simulink model "test_MartFracTransf_03_paper"  (Simulink 7.1)
settings: Solver=ode23tb  StartTime=0.0  StopTime=1  FixedStep=1e-6  MaxStep=1e-4  RelTol=1e-3
settings Model: Creator=Vagner  LastModifiedBy=Vagner
settings DebuggingCC: AlgebraicLoopMsg=none  SolverPrmCheckMsg=none

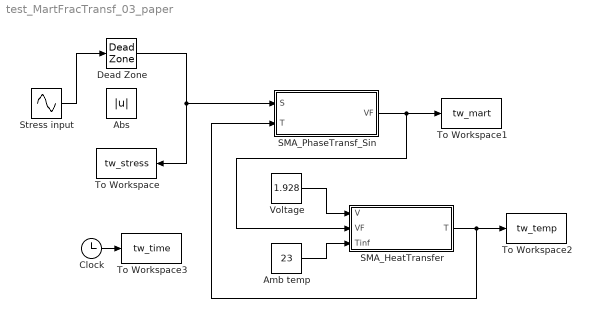
== system test_MartFracTransf_03_paper ==
  Abs : Abs  OutDataType=sfix(16)  OutScaling=2^0
  Amb temp : Constant  Value=23  OutDataType=sfix(16)  OutScaling=2^0
  Clock : Clock
      settings: Decimation=10
  Dead Zone : DeadZone  LowerValue=-inf  UpperValue=0  SaturateOnIntegerOverflow=on
  SMA_HeatTransfer : Subsystem  mask{varm=1.18e-3, varL=6025, varCp=350, varRA=0.7246, varRM=0.8197, varhc=150, varAc=977e-6, varT0=58.0049}
      mask prompts: varm "Spring mass [kg]"; varL "Latent heat [J / kg degC]"; varCp "Specific heat [J / kg degC]"; varRA "Electrical resistance of austenite [Ohm]"; varRM "Electrical resistance of martensite [Ohm]"; varhc "Convective heat transfer coefficient [J / m^2 degC s]"; varAc "Spring circunferential area [m^2]"; varT0 "Spring initial temperature [degC]"
      mask help: Mask parameters are some of the coefficients of equation (17) in Hadi et al. (2010). Commonly varying parameters are provided by input ports.
      mask init:
      | % when 'OK' or 'Apply' is clicked.
      | 
      | Hadi10_Temperature_InitMask(gcb);
      mask Help:
      | m: spring mass
      | L: latent heat
      | Cp: specific heat
      | RA: resistance in fully austenitic phase
      | RM: resistance in fully martensitic phase
      | hc: convective heat transfer coefficient
      | Ac: spring circunferential area
      | T0: spring initial temperature
      | 
      | Inputs:
      | V: voltage
      | VF: martensite volumetric fraction
      | Tinf: ambient temperature
      | 
      | Output:
      | T: spring temperature
      mask CallbackString: % Hadi10_Temperature_callback('Hadi10_Temperature_varm', gcb);|% Hadi10_Temperature_callback('Hadi10_Temperature_varL', gcb);|% Hadi10_Temperature_callback('Hadi10_Temperature_varCp', gcb);|% Hadi10_Temperature_callback('Hadi10_Temperature_varRA', gcb);|% Hadi10_Temperature_callback('Hadi10_Temperature_varRM', gcb);|% Hadi10_Temperature_callback('Hadi10_Temperature_varhc', gcb);|% Hadi10_Temperature_callback('Hadi10_Temperature_varAc', gcb);|% Hadi10_Temperature_callback('Hadi10_Temperature_varT0', gcb);
  SMA_PhaseTransf_Sin : Subsystem  mask{varCM=4, varCA=6, varSsmin=100, varSfmin=170, varMs=42, varAs=43, varAf=58}
      mask prompts: varCM "Forward stress-temperature slope (CM)"; varCA "Reverse stress-temperature slope (CA)"; varSsmin "Minimum stress for onset of forward transformation (Ssmin)"; varSfmin "Minimum stress for completion of forward transformation (Sfmin)"; varMs "Martensite start temperature (Ms)"; varAs "Austenite start temperature (As)"; varAf "Austenite finish temperature (Af)"
      mask init:
      | % when 'OK' or 'Apply' is clicked
      | 
      | SMA_PhaseTransf_Sin_InitMask(gcb);
  Stress input : Sin  Amplitude=600  Frequency=2*pi*1  SampleTime=0
  To Workspace : ToWorkspace  VariableName=tw_stress  SampleTime=-1  SaveFormat=Array
  To Workspace1 : ToWorkspace  VariableName=tw_mart  SampleTime=-1  SaveFormat=Array
  To Workspace2 : ToWorkspace  VariableName=tw_temp  SampleTime=-1  SaveFormat=Array
  To Workspace3 : ToWorkspace  VariableName=tw_time  SampleTime=-1  SaveFormat=Array
  Voltage : Constant  Value=1.928  OutDataType=sfix(16)  OutScaling=2^0
  wires:
  SMA_PhaseTransf_Sin/1(VF) -> To Workspace1/1, SMA_HeatTransfer/2(VF)
  SMA_HeatTransfer/1(T) -> To Workspace2/1, SMA_PhaseTransf_Sin/2(T)
  Voltage/1 -> SMA_HeatTransfer/1(V)
  Amb temp/1 -> SMA_HeatTransfer/3(Tinf)
  Clock/1 -> To Workspace3/1
  Dead Zone/1 -> SMA_PhaseTransf_Sin/1(S), To Workspace/1
  Stress input/1 -> Dead Zone/1

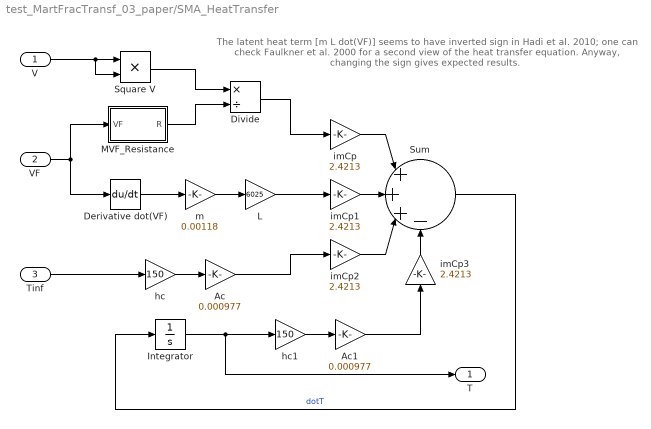
== system test_MartFracTransf_03_paper/SMA_HeatTransfer ==
  note: The latent heat term [m L dot(VF)] seems to
      | have inverted sign in Hadi et al. 2010; one
      | can check Faulkner et al. 2000 for a second
      | view of the heat transfer equation. Anyway,
      | changing the sign gives expected results.
  V : Inport  OutDataType=sfix(16)  OutScaling=2^0
  VF : Inport  Port=2  OutDataType=sfix(16)  OutScaling=2^0
  Tinf : Inport  Port=3  OutDataType=sfix(16)  OutScaling=2^0
  Ac : Gain  Gain=0.000977  ParameterDataType=sfix(16)  ParameterScaling=2^0  OutDataType=sfix(16)  OutScaling=2^0
  Ac1 : Gain  Gain=0.000977  ParameterDataType=sfix(16)  ParameterScaling=2^0  OutDataType=sfix(16)  OutScaling=2^0
  Derivative dot(VF) : Derivative
  Divide : Product  Inputs=*/  OutDataType=sfix(16)  OutScaling=2^-10
  Integrator : Integrator  InitialCondition=58.0049
  L : Gain  Gain=6025  ParameterDataType=sfix(16)  ParameterScaling=2^0  OutDataType=sfix(16)  OutScaling=2^0
  MVF_Resistance : Subsystem  mask{varRM=0.8197, varRA=0.7246}
      mask prompts: varRM "Fully-martensitic resistance [Ohm]"; varRA "Fully-austenitic resistance [Ohm]"
      mask help: Computes the electrical resistance as function of the martensitic fraction.
      mask init:
      | % when 'OK' or 'Apply' is clicked
      | 
      | MVF_Resistance_InitMask(gcb);
      mask Help:
      | DM: Fully-martensitic electrical resistance (in Ohms)
      | DA: Fully-austenitic elastic modulus (in Ohms)
      | 
      | The linear relation is assumed:
      | R = RA + VF(RM - RA)
      mask Display:
      | port_label('input', 1, 'VF');
      | port_label('output', 1, 'R');
  Square V : Product  OutDataType=sfix(16)  OutScaling=2^0  RndMeth=Zero
  Sum : Sum  Inputs=|+++-  OutDataType=sfix(16)  OutScaling=2^0
  hc : Gain  Gain=150  ParameterDataType=sfix(16)  ParameterScaling=2^0  OutDataType=sfix(16)  OutScaling=2^0
  hc1 : Gain  Gain=150  ParameterDataType=sfix(16)  ParameterScaling=2^0  OutDataType=sfix(16)  OutScaling=2^0
  imCp : Gain  Gain=2.4213  ParameterDataType=sfix(16)  ParameterScaling=2^0  OutDataType=sfix(16)  OutScaling=2^0
  imCp1 : Gain  Gain=2.4213  ParameterDataType=sfix(16)  ParameterScaling=2^0  OutDataType=sfix(16)  OutScaling=2^0
  imCp2 : Gain  Gain=2.4213  ParameterDataType=sfix(16)  ParameterScaling=2^0  OutDataType=sfix(16)  OutScaling=2^0
  imCp3 : Gain  Orientation=up  Gain=2.4213  ParameterDataType=sfix(16)  ParameterScaling=2^0  OutDataType=sfix(16)  OutScaling=2^0
  m : Gain  Gain=0.00118  ParameterDataType=sfix(16)  ParameterScaling=2^0  OutDataType=sfix(16)  OutScaling=2^0
  T : Outport  OutDataType=sfix(16)  OutScaling=2^0
  wires:
  V/1 -> Square V/1, Square V/2
  Square V/1 -> Divide/1
  MVF_Resistance/1(R) -> Divide/2
  Divide/1 -> imCp/1
  VF/1 -> Derivative dot(VF)/1, MVF_Resistance/1(VF)
  Derivative dot(VF)/1 -> m/1
  m/1 -> L/1
  L/1 -> imCp1/1
  hc/1 -> Ac/1
  Tinf/1 -> hc/1
  Ac/1 -> imCp2/1
  hc1/1 -> Ac1/1
  imCp/1 -> Sum/1
  imCp2/1 -> Sum/3
  imCp1/1 -> Sum/2
  Integrator/1 -> hc1/1, T/1
  Ac1/1 -> imCp3/1
  imCp3/1 -> Sum/4
  Sum/1 -> Integrator/1  "dotT"

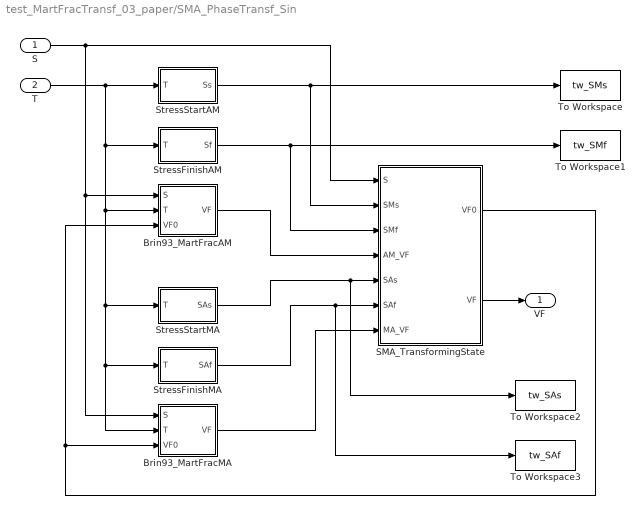
== system test_MartFracTransf_03_paper/SMA_PhaseTransf_Sin ==
  S : Inport  OutDataType=sfix(16)  OutScaling=2^0
  T : Inport  Port=2  OutDataType=sfix(16)  OutScaling=2^0
  Brin93_MartFracAM : Subsystem  mask{varSsmin=100, varSfmin=170, varCM=4, varMs=42}
      mask prompts: varSsmin "Minimum start stress"; varSfmin "Minimum finish stress"; varCM "Forward stress-temperature slope"; varMs "Martensite start temperature"
      mask init:
      | % when 'OK' or 'Apply' is clicked.
      | 
      | Brin93_MartFracAM_InitMask(gcb);
  Brin93_MartFracMA : Subsystem  mask{varCA=6, varAs=43, varAf=58}
      mask prompts: varCA "Reverse stress-temperature slope"; varAs "Austenite start temperature"; varAf "Austenite finish temperature"
      mask init:
      | % when 'OK' or 'Apply' is clicked.
      | 
      | Brin93_MartFracMA_InitMask(gcb);
  SMA_TransformingState : Subsystem
  StressFinishAM : Subsystem  mask{varCM=4, varSfmin=170, varMs=42}
      mask prompts: varCM "Forward stress-temperature slope"; varSfmin "Minimum stress for completion of transformation"; varMs "Martensite start temperature"
      mask help: Computes the critical stress for the completion of forward transformation.
      mask init:
      | % when 'OK' or 'Apply' is clicked
      | 
      | StressFinishAM_InitMask(gcb);
      mask Help:
      | Sf = Sfmin + CM * (T - Ms)
      | 
      | Sf: martensite finish stress
      | Sfmin: minimum finish stress (below Ms)
      | Ms: martensite start temperature
      | T: temperature
      mask Display:
      | port_label('input', 1, 'T');
      | port_label('output', 1, 'SMf');
  StressFinishMA : Subsystem  mask{varCA=6, varAf=58}
      mask prompts: varCA "Reverse stress-temperature slope"; varAf "Austenite finish temperature"
      mask help: Computes the critical stress for the completion of reverse transformation.
      mask init:
      | % when 'OK' or 'Apply' is clicked
      | 
      | StressFinishMA_InitMask(gcb);
      mask Help:
      | Sf = CA * (T - Af)
      | 
      | Ss: austenite finish stress
      | CA: stress-temperature slope
      | Af: austenite finish temperature
      | T: temperature
      mask Display:
      | port_label('input', 1, 'T');
      | port_label('output', 1, 'SAf');
  StressStartAM : Subsystem  mask{varCM=4, varSsmin=100, varMs=42}
      mask prompts: varCM "Forward stress-temperature slope"; varSsmin "Minimum stress for onset of transformation"; varMs "Martensite start temperature"
      mask help: Computes the critical stress for the onset of forward transformation.
      mask init:
      | % when 'OK' or 'Apply' is clicked
      | 
      | StressStartAM_InitMask(gcb);
      mask Help:
      | Ss = Ssmin + CM * (T - Ms)
      | 
      | Ss: martensite start stress
      | Ssmin: minimum start stress (below Ms)
      | Ms: martensite start temperature
      | T: temperature
      mask Display:
      | port_label('input', 1, 'T');
      | port_label('output', 1, 'SMs');
  StressStartMA : Subsystem  mask{varCA=6, varAs=43}
      mask prompts: varCA "Reverse stress-temperature slope"; varAs "Austenite start temperature"
      mask help: Computes the critical stress for the onset of reverse transformation.
      mask init:
      | % when 'OK' or 'Apply' is clicked
      | 
      | StressStartMA_InitMask(gcb);
      mask Help:
      | Ss = CA * (T - Ms)
      | 
      | Ss: austenite start stress
      | CA: stress-temperature slope
      | As: austenite start temperature
      | T: temperature
      mask Display:
      | port_label('input', 1, 'T');
      | port_label('output', 1, 'SAs');
  To Workspace : ToWorkspace  VariableName=tw_SMs  SampleTime=-1  SaveFormat=Array
  To Workspace1 : ToWorkspace  VariableName=tw_SMf  SampleTime=-1  SaveFormat=Array
  To Workspace2 : ToWorkspace  VariableName=tw_SAs  SampleTime=-1  SaveFormat=Array
  To Workspace3 : ToWorkspace  VariableName=tw_SAf  SampleTime=-1  SaveFormat=Array
  VF : Outport  OutDataType=sfix(16)  OutScaling=2^0
  wires:
  Brin93_MartFracMA/1(VF) -> SMA_TransformingState/7(MA_VF)
  Brin93_MartFracAM/1(VF) -> SMA_TransformingState/4(AM_VF)
  SMA_TransformingState/1(VF0) -> Brin93_MartFracMA/3(VF0), Brin93_MartFracAM/3(VF0)
  SMA_TransformingState/2(VF) -> VF/1
  StressFinishMA/1(SAf) -> SMA_TransformingState/6(SAf), To Workspace3/1
  StressStartMA/1(SAs) -> SMA_TransformingState/5(SAs), To Workspace2/1
  T/1 -> Brin93_MartFracAM/2(T), Brin93_MartFracMA/2(T), StressFinishMA/1(T), StressStartMA/1(T), StressFinishAM/1(T), StressStartAM/1(T)
  S/1 -> Brin93_MartFracMA/1(S), Brin93_MartFracAM/1(S), SMA_TransformingState/1(S)
  StressFinishAM/1(Sf) -> SMA_TransformingState/3(SMf), To Workspace1/1
  StressStartAM/1(Ss) -> SMA_TransformingState/2(SMs), To Workspace/1

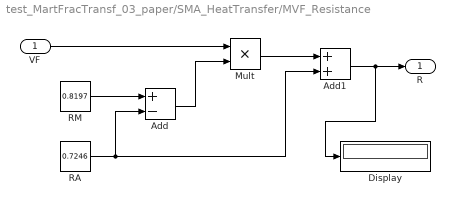
== system test_MartFracTransf_03_paper/SMA_HeatTransfer/MVF_Resistance ==
  VF : Inport  OutDataType=sfix(16)  OutScaling=2^0
  Add : Sum  Inputs=+-  OutDataType=sfix(16)  OutScaling=2^-10
  Add1 : Sum  OutDataType=sfix(16)  OutScaling=2^-10
  Display : Display
  Mult : Product  Inputs=**  OutDataType=sfix(16)  OutScaling=2^-10
  RA : Constant  Value=0.7246  OutDataType=sfix(16)  OutScaling=2^0
  RM : Constant  Value=0.8197  OutDataType=sfix(16)  OutScaling=2^0
  R : Outport  OutDataType=sfix(16)  OutScaling=2^0
  wires:
  RA/1 -> Add1/2, Add/2
  RM/1 -> Add/1
  Add1/1 -> Display/1, R/1
  Mult/1 -> Add1/1
  Add/1 -> Mult/2
  VF/1 -> Mult/1

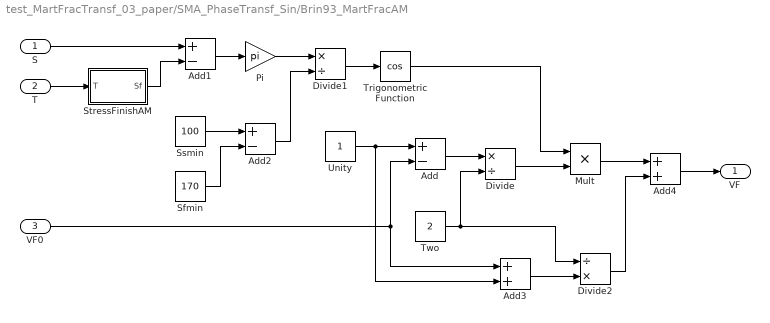
== system test_MartFracTransf_03_paper/SMA_PhaseTransf_Sin/Brin93_MartFracAM ==
  S : Inport  OutDataType=sfix(16)  OutScaling=2^0
  T : Inport  Port=2  OutDataType=sfix(16)  OutScaling=2^0
  VF0 : Inport  Port=3  OutDataType=sfix(16)  OutScaling=2^0
  Add : Sum  Inputs=+-  OutDataType=sfix(16)  OutScaling=2^-10
  Add1 : Sum  Inputs=+-  OutDataType=sfix(16)  OutScaling=2^-10
  Add2 : Sum  Inputs=+-  OutDataType=sfix(16)  OutScaling=2^-10
  Add3 : Sum  OutDataType=sfix(16)  OutScaling=2^-10
  Add4 : Sum  OutDataType=sfix(16)  OutScaling=2^-10
  Divide : Product  Inputs=*/  OutDataType=sfix(16)  OutScaling=2^-10
  Divide1 : Product  Inputs=*/  OutDataType=sfix(16)  OutScaling=2^-10
  Divide2 : Product  Inputs=/*  OutDataType=sfix(16)  OutScaling=2^-10
  Mult : Product  Inputs=**  OutDataType=sfix(16)  OutScaling=2^-10
  Pi : Gain  Gain=pi  ParameterDataType=sfix(16)  ParameterScaling=2^0  OutDataType=sfix(16)  OutScaling=2^0
  Sfmin : Constant  Value=170  OutDataType=sfix(16)  OutScaling=2^0
  Ssmin : Constant  Value=100  OutDataType=sfix(16)  OutScaling=2^0
  StressFinishAM : Subsystem  mask{varCM=4, varSfmin=170, varMs=42}
      mask prompts: varCM "Forward stress-temperature slope"; varSfmin "Minimum stress for completion of transformation"; varMs "Martensite start temperature"
      mask help: Computes the critical stress for the completion of forward transformation.
      mask init:
      | % when 'OK' or 'Apply' is clicked
      | 
      | StressFinishAM_InitMask(gcb);
      mask Help:
      | Sf = Sfmin + CM * (T - Ms)
      | 
      | Sf: martensite finish stress
      | Sfmin: minimum finish stress (below Ms)
      | Ms: martensite start temperature
      | T: temperature
      mask Display:
      | port_label('input', 1, 'T');
      | port_label('output', 1, 'SMf');
  Trigonometric Function : Trigonometry  Operator=cos
  Two : Constant  Value=2  OutDataType=sfix(16)  OutScaling=2^0
  Unity : Constant  OutDataType=sfix(16)  OutScaling=2^0
  VF : Outport  OutDataType=sfix(16)  OutScaling=2^0
  wires:
  Add3/1 -> Divide2/2
  Trigonometric Function/1 -> Mult/1
  Divide/1 -> Mult/2
  Add4/1 -> VF/1
  Divide2/1 -> Add4/2
  Mult/1 -> Add4/1
  Divide1/1 -> Trigonometric Function/1
  Add2/1 -> Divide1/2
  Sfmin/1 -> Add2/2
  Ssmin/1 -> Add2/1
  Pi/1 -> Divide1/1
  Add1/1 -> Pi/1
  StressFinishAM/1(Sf) -> Add1/2
  S/1 -> Add1/1
  Two/1 -> Divide2/1, Divide/2
  Add/1 -> Divide/1
  VF0/1 -> Add3/1, Add/2
  Unity/1 -> Add3/2, Add/1
  T/1 -> StressFinishAM/1(T)

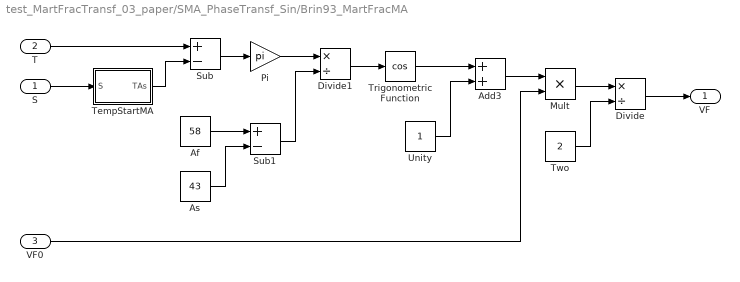
== system test_MartFracTransf_03_paper/SMA_PhaseTransf_Sin/Brin93_MartFracMA ==
  S : Inport  OutDataType=sfix(16)  OutScaling=2^0
  T : Inport  Port=2  OutDataType=sfix(16)  OutScaling=2^0
  VF0 : Inport  Port=3  OutDataType=sfix(16)  OutScaling=2^0
  Add3 : Sum  OutDataType=sfix(16)  OutScaling=2^-10
  Af : Constant  Value=58  OutDataType=sfix(16)  OutScaling=2^0
  As : Constant  Value=43  OutDataType=sfix(16)  OutScaling=2^0
  Divide : Product  Inputs=*/  OutDataType=sfix(16)  OutScaling=2^-10
  Divide1 : Product  Inputs=*/  OutDataType=sfix(16)  OutScaling=2^-10
  Mult : Product  Inputs=**  OutDataType=sfix(16)  OutScaling=2^-10
  Pi : Gain  Gain=pi  ParameterDataType=sfix(16)  ParameterScaling=2^0  OutDataType=sfix(16)  OutScaling=2^0
  Sub : Sum  Inputs=+-  OutDataType=sfix(16)  OutScaling=2^-10
  Sub1 : Sum  Inputs=+-  OutDataType=sfix(16)  OutScaling=2^-10
  TempStartMA : Subsystem  mask{varCA=6, varAs=43}
      mask prompts: varCA "Reverse stress-temperature slope"; varAs "Austenite start temperature"
      mask help: Computes the critical temperature for the onset of reverse transformation (for non-zero stress).
      mask init:
      | % when 'OK' or 'Apply' is clicked
      | 
      | TempStartMA_InitMask(gcb);
      mask Help:
      | TAs = As + S / CA
      | 
      | TAs: austenite start temperature (for S > 0)
      | CA: stress-temperature slope
      | As: austenite start temperature
      mask Display:
      | port_label('input', 1, 'S');
      | port_label('output', 1, 'TAs');
  Trigonometric Function : Trigonometry  Operator=cos
  Two : Constant  Value=2  OutDataType=sfix(16)  OutScaling=2^0
  Unity : Constant  OutDataType=sfix(16)  OutScaling=2^0
  VF : Outport  OutDataType=sfix(16)  OutScaling=2^0
  wires:
  VF0/1 -> Mult/2
  Divide/1 -> VF/1
  Add3/1 -> Mult/1
  Trigonometric Function/1 -> Add3/1
  Unity/1 -> Add3/2
  Two/1 -> Divide/2
  Mult/1 -> Divide/1
  S/1 -> TempStartMA/1(S)
  T/1 -> Sub/1
  TempStartMA/1(TAs) -> Sub/2
  Sub/1 -> Pi/1
  Pi/1 -> Divide1/1
  Af/1 -> Sub1/1
  As/1 -> Sub1/2
  Sub1/1 -> Divide1/2
  Divide1/1 -> Trigonometric Function/1

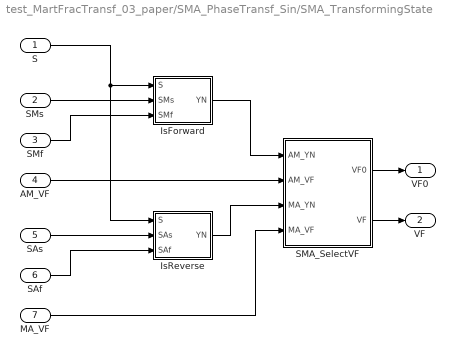
== system test_MartFracTransf_03_paper/SMA_PhaseTransf_Sin/SMA_TransformingState ==
  S : Inport
  SMs : Inport  Port=2
  SMf : Inport  Port=3
  AM_VF : Inport  Port=4
  SAs : Inport  Port=5
  SAf : Inport  Port=6
  MA_VF : Inport  Port=7
  IsForward : Subsystem
  IsReverse : Subsystem
  SMA_SelectVF : Subsystem
  VF0 : Outport
  VF : Outport  Port=2
  wires:
  MA_VF/1 -> SMA_SelectVF/4(MA_VF)
  SMA_SelectVF/2(VF) -> VF/1
  IsReverse/1(YN) -> SMA_SelectVF/3(MA_YN)
  SMA_SelectVF/1(VF0) -> VF0/1
  AM_VF/1 -> SMA_SelectVF/2(AM_VF)
  IsForward/1(YN) -> SMA_SelectVF/1(AM_YN)
  SAf/1 -> IsReverse/3(SAf)
  SAs/1 -> IsReverse/2(SAs)
  SMf/1 -> IsForward/3(SMf)
  SMs/1 -> IsForward/2(SMs)
  S/1 -> IsReverse/1(S), IsForward/1(S)

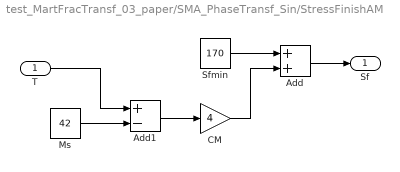
== system test_MartFracTransf_03_paper/SMA_PhaseTransf_Sin/StressFinishAM ==
  T : Inport  OutDataType=sfix(16)  OutScaling=2^0
  Add : Sum  OutDataType=sfix(16)  OutScaling=2^-10
  Add1 : Sum  Inputs=+-  OutDataType=sfix(16)  OutScaling=2^-10
  CM : Gain  Gain=4  ParameterDataType=sfix(16)  ParameterScaling=2^0  OutDataType=sfix(16)  OutScaling=2^0
  Ms : Constant  Value=42  OutDataType=sfix(16)  OutScaling=2^0
  Sfmin : Constant  Value=170  OutDataType=sfix(16)  OutScaling=2^0
  Sf : Outport  OutDataType=sfix(16)  OutScaling=2^0
  wires:
  Sfmin/1 -> Add/1
  T/1 -> Add1/1
  Ms/1 -> Add1/2
  Add1/1 -> CM/1
  CM/1 -> Add/2
  Add/1 -> Sf/1

== system test_MartFracTransf_03_paper/SMA_PhaseTransf_Sin/StressFinishMA ==
  T : Inport  OutDataType=sfix(16)  OutScaling=2^0
  Add1 : Sum  Inputs=+-  OutDataType=sfix(16)  OutScaling=2^-10
  Af : Constant  Value=58  OutDataType=sfix(16)  OutScaling=2^0
  CA : Gain  Gain=6  ParameterDataType=sfix(16)  ParameterScaling=2^0  OutDataType=sfix(16)  OutScaling=2^0
  SAf : Outport  OutDataType=sfix(16)  OutScaling=2^0
  wires:
  CA/1 -> SAf/1
  Add1/1 -> CA/1
  Af/1 -> Add1/2
  T/1 -> Add1/1

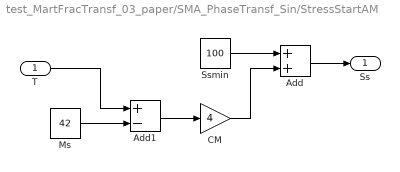
== system test_MartFracTransf_03_paper/SMA_PhaseTransf_Sin/StressStartAM ==
  T : Inport  OutDataType=sfix(16)  OutScaling=2^0
  Add : Sum  OutDataType=sfix(16)  OutScaling=2^-10
  Add1 : Sum  Inputs=+-  OutDataType=sfix(16)  OutScaling=2^-10
  CM : Gain  Gain=4  ParameterDataType=sfix(16)  ParameterScaling=2^0  OutDataType=sfix(16)  OutScaling=2^0
  Ms : Constant  Value=42  OutDataType=sfix(16)  OutScaling=2^0
  Ssmin : Constant  Value=100  OutDataType=sfix(16)  OutScaling=2^0
  Ss : Outport  OutDataType=sfix(16)  OutScaling=2^0
  wires:
  Add/1 -> Ss/1
  CM/1 -> Add/2
  Add1/1 -> CM/1
  Ms/1 -> Add1/2
  T/1 -> Add1/1
  Ssmin/1 -> Add/1

== system test_MartFracTransf_03_paper/SMA_PhaseTransf_Sin/StressStartMA ==
  T : Inport  OutDataType=sfix(16)  OutScaling=2^0
  Add1 : Sum  Inputs=+-  OutDataType=sfix(16)  OutScaling=2^-10
  As : Constant  Value=43  OutDataType=sfix(16)  OutScaling=2^0
  CA : Gain  Gain=6  ParameterDataType=sfix(16)  ParameterScaling=2^0  OutDataType=sfix(16)  OutScaling=2^0
  SAs : Outport  OutDataType=sfix(16)  OutScaling=2^0
  wires:
  CA/1 -> SAs/1
  T/1 -> Add1/1
  As/1 -> Add1/2
  Add1/1 -> CA/1

== system test_MartFracTransf_03_paper/SMA_PhaseTransf_Sin/Brin93_MartFracAM/StressFinishAM ==
  T : Inport  OutDataType=sfix(16)  OutScaling=2^0
  Add : Sum  OutDataType=sfix(16)  OutScaling=2^-10
  Add1 : Sum  Inputs=+-  OutDataType=sfix(16)  OutScaling=2^-10
  CM : Gain  Gain=4  ParameterDataType=sfix(16)  ParameterScaling=2^0  OutDataType=sfix(16)  OutScaling=2^0
  Ms : Constant  Value=42  OutDataType=sfix(16)  OutScaling=2^0
  Sfmin : Constant  Value=170  OutDataType=sfix(16)  OutScaling=2^0
  Sf : Outport  OutDataType=sfix(16)  OutScaling=2^0
  wires:
  Sfmin/1 -> Add/1
  T/1 -> Add1/1
  Ms/1 -> Add1/2
  Add1/1 -> CM/1
  CM/1 -> Add/2
  Add/1 -> Sf/1

== system test_MartFracTransf_03_paper/SMA_PhaseTransf_Sin/Brin93_MartFracMA/TempStartMA ==
  S : Inport  OutDataType=sfix(16)  OutScaling=2^0
  Add : Sum  OutDataType=sfix(16)  OutScaling=2^-10
  As : Constant  Value=43  OutDataType=sfix(16)  OutScaling=2^0
  CA : Constant  Value=6  OutDataType=sfix(16)  OutScaling=2^0
  Divide : Product  Inputs=*/  OutDataType=sfix(16)  OutScaling=2^-10
  TAs : Outport  OutDataType=sfix(16)  OutScaling=2^0
  wires:
  Add/1 -> TAs/1
  Divide/1 -> Add/1
  CA/1 -> Divide/2
  S/1 -> Divide/1
  As/1 -> Add/2

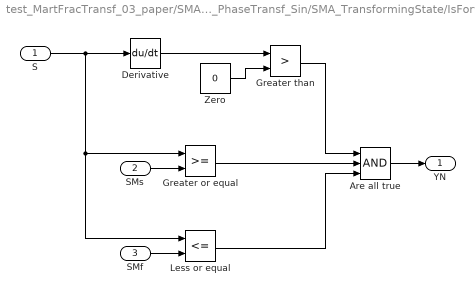
== system test_MartFracTransf_03_paper/SMA_PhaseTransf_Sin/SMA_TransformingState/IsForward ==
  S : Inport  OutDataType=sfix(16)  OutScaling=2^0
  SMs : Inport  Port=2  OutDataType=sfix(16)  OutScaling=2^0
  SMf : Inport  Port=3  OutDataType=sfix(16)  OutScaling=2^0
  Are all true : Logic  Inputs=3  AllPortsSameDT=off  OutDataTypeMode=boolean  OutDataTypeStr=boolean
  Derivative : Derivative
  Greater or equal : RelationalOperator  LogicOutDataTypeMode=boolean  OutDataTypeStr=boolean
  Greater than : RelationalOperator  Operator=>  LogicOutDataTypeMode=boolean  OutDataTypeStr=boolean
  Less or equal : RelationalOperator  Operator=<=  LogicOutDataTypeMode=boolean  OutDataTypeStr=boolean
  Zero : Constant  Value=0  OutDataType=sfix(16)  OutScaling=2^0
  YN : Outport  OutDataType=sfix(16)  OutScaling=2^0
  wires:
  Are all true/1 -> YN/1
  Less or equal/1 -> Are all true/3
  Greater or equal/1 -> Are all true/2
  Greater than/1 -> Are all true/1
  SMf/1 -> Less or equal/2
  SMs/1 -> Greater or equal/2
  Derivative/1 -> Greater than/1
  Zero/1 -> Greater than/2
  S/1 -> Less or equal/1, Greater or equal/1, Derivative/1

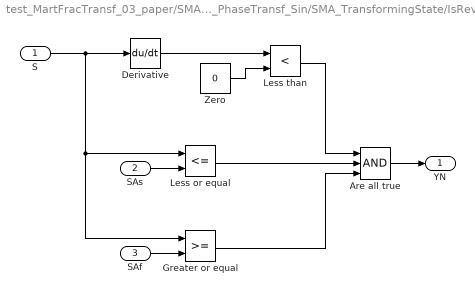
== system test_MartFracTransf_03_paper/SMA_PhaseTransf_Sin/SMA_TransformingState/IsReverse ==
  S : Inport  OutDataType=sfix(16)  OutScaling=2^0
  SAs : Inport  Port=2  OutDataType=sfix(16)  OutScaling=2^0
  SAf : Inport  Port=3  OutDataType=sfix(16)  OutScaling=2^0
  Are all true : Logic  Inputs=3  AllPortsSameDT=off  OutDataTypeMode=boolean  OutDataTypeStr=boolean
  Derivative : Derivative
  Greater or equal : RelationalOperator  LogicOutDataTypeMode=boolean  OutDataTypeStr=boolean
  Less than : RelationalOperator  Operator=<  LogicOutDataTypeMode=boolean  OutDataTypeStr=boolean
  Less or equal : RelationalOperator  Operator=<=  LogicOutDataTypeMode=boolean  OutDataTypeStr=boolean
  Zero : Constant  Value=0  OutDataType=sfix(16)  OutScaling=2^0
  YN : Outport  OutDataType=sfix(16)  OutScaling=2^0
  wires:
  S/1 -> Derivative/1, Less or equal/1, Greater or equal/1
  Zero/1 -> Less than/2
  Derivative/1 -> Less than/1
  SAs/1 -> Less or equal/2
  SAf/1 -> Greater or equal/2
  Less than/1 -> Are all true/1
  Less or equal/1 -> Are all true/2
  Greater or equal/1 -> Are all true/3
  Are all true/1 -> YN/1

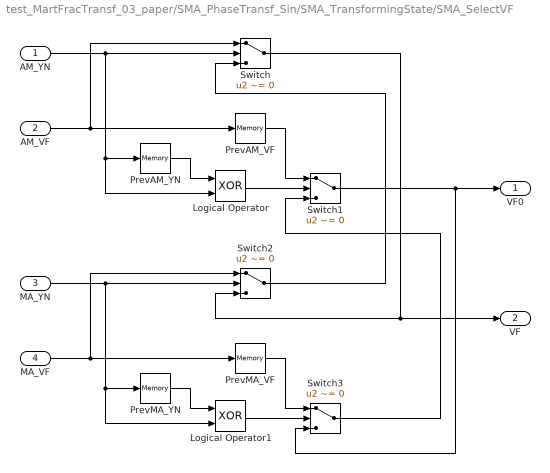
== system test_MartFracTransf_03_paper/SMA_PhaseTransf_Sin/SMA_TransformingState/SMA_SelectVF ==
  AM_YN : Inport
  AM_VF : Inport  Port=2
  MA_YN : Inport  Port=3
  MA_VF : Inport  Port=4
  Logical Operator : Logic  Operator=XOR  AllPortsSameDT=off  OutDataTypeMode=boolean  OutDataTypeStr=boolean
  Logical Operator1 : Logic  Operator=XOR  AllPortsSameDT=off  OutDataTypeMode=boolean  OutDataTypeStr=boolean
  PrevAM_VF : Memory
  PrevAM_YN : Memory
  PrevMA_VF : Memory
  PrevMA_YN : Memory
  Switch{,1..3} (4 alike) : Switch  Criteria=u2 ~= 0  OutDataType=sfix(16)  OutScaling=2^0
  VF0 : Outport
  VF : Outport  Port=2
  wires:
  PrevAM_YN/1 -> Logical Operator/1
  PrevMA_YN/1 -> Logical Operator1/1
  MA_VF/1 -> PrevMA_VF/1, Switch2/1
  Switch3/1 -> Switch1/3
  PrevMA_VF/1 -> Switch3/1
  Logical Operator1/1 -> Switch3/2
  Switch2/1 -> Switch/3
  MA_YN/1 -> PrevMA_YN/1, Logical Operator1/2, Switch2/2
  AM_VF/1 -> PrevAM_VF/1, Switch/1
  Switch1/1 -> VF0/1, Switch3/3
  PrevAM_VF/1 -> Switch1/1
  Logical Operator/1 -> Switch1/2
  Switch/1 -> VF/1, Switch2/3
  AM_YN/1 -> PrevAM_YN/1, Logical Operator/2, Switch/2
